simulink model "volo_radio_controller"  (Simulink 8.0)
settings: Solver=ode45  SolverMode=SingleTasking  StartTime=0.0  StopTime=1000  RelTol=1e-3
InitFcn:
  | volo_radio_controller_init
values from neighbouring files (symbols this model uses):
  cFI = fi(cMult, 1, 13, 11)    [volo_radio_controller_init.m]
  gFI = fi(gain, 1, 13, 11)    [volo_radio_controller_init.m]
  sFI = fi(sMult, 1, 13, 11)    [volo_radio_controller_init.m]
undefined symbols (not defined in the file or in its folder): gcbh, xlBlockLoadCallback, xlGetNormalizedPeriod, xlipgetpartsetting
libraries: xbsIndex_r4 x380, xbsEDKLib_r4 x1
(part 4 of 5)

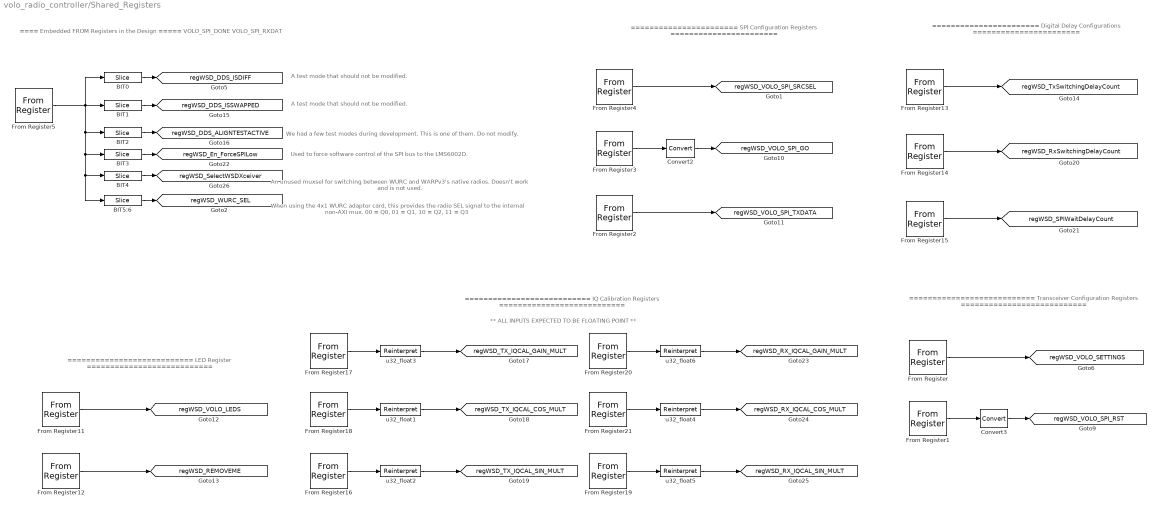
== system volo_radio_controller/Shared_Registers ==
  note: A test mode that should not be modified.
  note: We had a few test modes during development. This is one of them. Do not modify.
  note: Used to force software control of the SPI bus to the LMS6002D.
  note: When using the 4x1 WURC adaptor card, this provides the radio SEL signal
      | to the internal non-AXI mux.  00 = Q0, 01 = Q1, 10 = Q2, 11 = Q3
  note: An unused muxsel for switching between WURC and WARPv3's native radios.
      | Doesn't work and is not used.
  note: ==== Embedded FROM Registers in the Design =====
      | VOLO_SPI_DONE
      | VOLO_SPI_RXDAT
  note: ===========================
      | LED Register
      | ===========================
  note: =======================
      | Digital Delay Configurations
      | =======================
  note: =======================
      | SPI Configuration Registers
      | =======================
  note: ===========================
      | Transceiver Configuration Registers
      | ===========================
  note: ===========================
      | IQ Calibration Registers
      | ===========================
  note: ** ALL INPUTS EXPECTED TO BE FLOATING POINT **
  note: A test mode that should not be modified.
  BIT0 : xbsIndex_r4/Slice  nbits=1  boolean_output=on  mode=Lower Bit Location + Width  bit1=0  base1=LSB of Input  bit0=0  base0=LSB of Input  dbl_ovrd=off  block_type=slice
  BIT1 : xbsIndex_r4/Slice  nbits=1  boolean_output=on  mode=Lower Bit Location + Width  bit1=0  base1=LSB of Input  bit0=1  base0=LSB of Input  dbl_ovrd=off  block_type=slice
  BIT2 : xbsIndex_r4/Slice  nbits=1  boolean_output=on  mode=Lower Bit Location + Width  bit1=0  base1=LSB of Input  bit0=2  base0=LSB of Input  dbl_ovrd=off  block_type=slice
  BIT3 : xbsIndex_r4/Slice  nbits=1  boolean_output=on  mode=Lower Bit Location + Width  bit1=0  base1=LSB of Input  bit0=3  base0=LSB of Input  dbl_ovrd=off  block_type=slice
  BIT4 : xbsIndex_r4/Slice  nbits=1  boolean_output=on  mode=Lower Bit Location + Width  bit1=0  base1=LSB of Input  bit0=4  base0=LSB of Input  dbl_ovrd=off  block_type=slice
  BIT5:6 : xbsIndex_r4/Slice  nbits=2  boolean_output=off  mode=Lower Bit Location + Width  bit1=0  base1=LSB of Input  bit0=5  base0=LSB of Input  dbl_ovrd=off  block_type=slice
  Convert2 : xbsIndex_r4/Convert  gui_display_data_type=Boolean  arith_type=Boolean  n_bits=32  bin_pt=0  float_type=Single  exp_bits=8  fraction_bits=24  quantization=Truncate  overflow=Wrap  en=off  latency=0  dbl_ovrd=off  pipeline=off  block_type=convert
  Convert3 : xbsIndex_r4/Convert  gui_display_data_type=Boolean  arith_type=Boolean  n_bits=32  bin_pt=0  float_type=Single  exp_bits=8  fraction_bits=24  quantization=Truncate  overflow=Wrap  en=off  latency=0  dbl_ovrd=off  pipeline=off  block_type=convert
  From Register : xbsIndex_r4/From Register  shared_memory_name='VOLO_SETTINGS'  init=15  period=1  ownership=Locally owned and initialized  gui_display_data_type=Fixed-point  arith_type=Unsigned  n_bits=32  bin_pt=0  preci_type=Single  dbl_ovrd=off  block_type=fromreg
      settings: AttributesFormatString=<< %<shared_memory_name> >>  infoedit="Register block that reads data to a shared memory register.  Delay of one sample period."
  From Register1 : xbsIndex_r4/From Register  shared_memory_name='VOLO_SPI_RST'  init=0  period=1  ownership=Locally owned and initialized  gui_display_data_type=Fixed-point  arith_type=Unsigned  n_bits=1  bin_pt=0  preci_type=Single  dbl_ovrd=off  block_type=fromreg
      settings: AttributesFormatString=<< %<shared_memory_name> >>  infoedit="Register block that reads data to a shared memory register.  Delay of one sample period."
  From Register11 : xbsIndex_r4/From Register  shared_memory_name='VOLO_LED'  init=0  period=1  ownership=Owned and initialized elsewhere  gui_display_data_type=Fixed-point  arith_type=Unsigned  n_bits=32  bin_pt=0  preci_type=Single  dbl_ovrd=off  block_type=fromreg
      settings: AttributesFormatString=<< %<shared_memory_name> >>  infoedit="Register block that reads data to a shared memory register.  Delay of one sample period."
  From Register12 : xbsIndex_r4/From Register  shared_memory_name='VOLO_ADAPTER_GPIO'  init=0  period=1  ownership=Owned and initialized elsewhere  gui_display_data_type=Fixed-point  arith_type=Unsigned  n_bits=32  bin_pt=0  preci_type=Single  dbl_ovrd=off  block_type=fromreg
      settings: AttributesFormatString=<< %<shared_memory_name> >>  infoedit="Register block that reads data to a shared memory register.  Delay of one sample period."
  From Register13 : xbsIndex_r4/From Register  shared_memory_name='WSD_SWITCHINGDELAYCOUNT'  init=0  period=1  ownership=Locally owned and initialized  gui_display_data_type=Fixed-point  arith_type=Unsigned  n_bits=32  bin_pt=0  preci_type=Single  dbl_ovrd=off  block_type=fromreg
      settings: AttributesFormatString=<< %<shared_memory_name> >>  infoedit="Register block that reads data to a shared memory register.  Delay of one sample period."
  From Register14 : xbsIndex_r4/From Register  shared_memory_name='WSD_RXSWITCHINGDELAYCOUNT'  init=0  period=1  ownership=Locally owned and initialized  gui_display_data_type=Fixed-point  arith_type=Unsigned  n_bits=32  bin_pt=0  preci_type=Single  dbl_ovrd=off  block_type=fromreg
      settings: AttributesFormatString=<< %<shared_memory_name> >>  infoedit="Register block that reads data to a shared memory register.  Delay of one sample period."
  From Register15 : xbsIndex_r4/From Register  shared_memory_name='WSD_SPIWAITDELAYCOUNT'  init=0  period=1  ownership=Locally owned and initialized  gui_display_data_type=Fixed-point  arith_type=Unsigned  n_bits=32  bin_pt=0  preci_type=Single  dbl_ovrd=off  block_type=fromreg
      settings: AttributesFormatString=<< %<shared_memory_name> >>  infoedit="Register block that reads data to a shared memory register.  Delay of one sample period."
  From Register16 : xbsIndex_r4/From Register  shared_memory_name='VOLO_TX_SIN_MULT'  init=str2num(sFI.dec)  period=2  ownership=Locally owned and initialized  gui_display_data_type=Fixed-point  arith_type=Unsigned  n_bits=32  bin_pt=0  preci_type=Single  dbl_ovrd=off  block_type=fromreg
      settings: AttributesFormatString=<< %<shared_memory_name> >>  infoedit="Register block that reads data to a shared memory register.  Delay of one sample period."
  From Register17 : xbsIndex_r4/From Register  shared_memory_name='VOLO_TX_GAIN_MULT'  init=str2num(gFI.dec)  period=2  ownership=Locally owned and initialized  gui_display_data_type=Fixed-point  arith_type=Unsigned  n_bits=32  bin_pt=0  preci_type=Single  dbl_ovrd=off  block_type=fromreg
      settings: AttributesFormatString=<< %<shared_memory_name> >>  infoedit="Register block that reads data to a shared memory register.  Delay of one sample period."
  From Register18 : xbsIndex_r4/From Register  shared_memory_name='VOLO_TX_COS_MULT'  init=str2num(cFI.dec)  period=2  ownership=Locally owned and initialized  gui_display_data_type=Fixed-point  arith_type=Unsigned  n_bits=32  bin_pt=0  preci_type=Single  dbl_ovrd=off  block_type=fromreg
      settings: AttributesFormatString=<< %<shared_memory_name> >>  infoedit="Register block that reads data to a shared memory register.  Delay of one sample period."
  From Register19 : xbsIndex_r4/From Register  shared_memory_name='VOLO_RX_SIN_MULT'  init=str2num(sFI.dec)  period=2  ownership=Locally owned and initialized  gui_display_data_type=Fixed-point  arith_type=Unsigned  n_bits=32  bin_pt=0  preci_type=Single  dbl_ovrd=off  block_type=fromreg
      settings: AttributesFormatString=<< %<shared_memory_name> >>  infoedit="Register block that reads data to a shared memory register.  Delay of one sample period."
  From Register2 : xbsIndex_r4/From Register  shared_memory_name='VOLO_SPI_TXDAT'  init=hex2dec('ADAD')  period=1  ownership=Locally owned and initialized  gui_display_data_type=Fixed-point  arith_type=Unsigned  n_bits=32  bin_pt=0  preci_type=Single  dbl_ovrd=off  block_type=fromreg
      settings: AttributesFormatString=<< %<shared_memory_name> >>  infoedit="Register block that reads data to a shared memory register.  Delay of one sample period."
  From Register20 : xbsIndex_r4/From Register  shared_memory_name='VOLO_RX_GAIN_MULT'  init=str2num(gFI.dec)  period=2  ownership=Locally owned and initialized  gui_display_data_type=Fixed-point  arith_type=Unsigned  n_bits=32  bin_pt=0  preci_type=Single  dbl_ovrd=off  block_type=fromreg
      settings: AttributesFormatString=<< %<shared_memory_name> >>  infoedit="Register block that reads data to a shared memory register.  Delay of one sample period."
  From Register21 : xbsIndex_r4/From Register  shared_memory_name='VOLO_RX_COS_MULT'  init=str2num(cFI.dec)  period=2  ownership=Locally owned and initialized  gui_display_data_type=Fixed-point  arith_type=Unsigned  n_bits=32  bin_pt=0  preci_type=Single  dbl_ovrd=off  block_type=fromreg
      settings: AttributesFormatString=<< %<shared_memory_name> >>  infoedit="Register block that reads data to a shared memory register.  Delay of one sample period."
  From Register3 : xbsIndex_r4/From Register  shared_memory_name='VOLO_SPI_GO'  init=1  period=1  ownership=Locally owned and initialized  gui_display_data_type=Fixed-point  arith_type=Unsigned  n_bits=1  bin_pt=0  preci_type=Single  dbl_ovrd=off  block_type=fromreg
      settings: AttributesFormatString=<< %<shared_memory_name> >>  infoedit="Register block that reads data to a shared memory register.  Delay of one sample period."
  From Register4 : xbsIndex_r4/From Register  shared_memory_name='VOLO_SPI_SRCSEL'  init=1  period=1  ownership=Locally owned and initialized  gui_display_data_type=Fixed-point  arith_type=Unsigned  n_bits=1  bin_pt=0  preci_type=Single  dbl_ovrd=off  block_type=fromreg
      settings: AttributesFormatString=<< %<shared_memory_name> >>  infoedit="Register block that reads data to a shared memory register.  Delay of one sample period."
  From Register5 : xbsIndex_r4/From Register  shared_memory_name='VOLO_CONTROLLER_CONFIG_R'  init=19  period=1  ownership=Locally owned and initialized  gui_display_data_type=Fixed-point  arith_type=Unsigned  n_bits=32  bin_pt=0  preci_type=Single  dbl_ovrd=off  block_type=fromreg
      settings: AttributesFormatString=<< %<shared_memory_name> >>  infoedit="Register block that reads data to a shared memory register.  Delay of one sample period."
  u32_float{1..6} (6 alike) : xbsIndex_r4/Reinterpret  force_arith_type=on  arith_type=Floating-point  force_bin_pt=on  bin_pt=24  block_type=reinterpret
  tag scope: regWSD_DDS_ALIGNTESTACTIVE=global, regWSD_DDS_ISDIFF=global, regWSD_DDS_ISSWAPPED=global, regWSD_En_ForceSPILow=global, regWSD_REMOVEME=global, regWSD_RX_IQCAL_COS_MULT=global, regWSD_RX_IQCAL_GAIN_MULT=global, regWSD_RX_IQCAL_SIN_MULT=global, regWSD_RxSwitchingDelayCount=global, regWSD_SPIWaitDelayCount=global, regWSD_SelectWSDXceiver=global, regWSD_TX_IQCAL_COS_MULT=global, regWSD_TX_IQCAL_GAIN_MULT=global, regWSD_TX_IQCAL_SIN_MULT=global, regWSD_TxSwitchingDelayCount=global, regWSD_VOLO_LEDS=global, regWSD_VOLO_SETTINGS=global, regWSD_VOLO_SPI_GO=global, regWSD_VOLO_SPI_RST=global, regWSD_VOLO_SPI_SRCSEL=global, regWSD_VOLO_SPI_TXDATA=global, regWSD_WURC_SEL=global
  wires:
  From Register/1 -> [regWSD_VOLO_SETTINGS]
  From Register1/1 -> Convert3/1
  Convert3/1 -> [regWSD_VOLO_SPI_RST]
  From Register4/1 -> [regWSD_VOLO_SPI_SRCSEL]
  From Register3/1 -> Convert2/1
  Convert2/1 -> [regWSD_VOLO_SPI_GO]
  From Register2/1 -> [regWSD_VOLO_SPI_TXDATA]
  BIT0/1 -> [regWSD_DDS_ISDIFF]
  From Register11/1 -> [regWSD_VOLO_LEDS]
  From Register12/1 -> [regWSD_REMOVEME]
  From Register17/1 -> u32_float3/1
  From Register18/1 -> u32_float1/1
  From Register16/1 -> u32_float2/1
  u32_float3/1 -> [regWSD_TX_IQCAL_GAIN_MULT]
  u32_float1/1 -> [regWSD_TX_IQCAL_COS_MULT]
  u32_float2/1 -> [regWSD_TX_IQCAL_SIN_MULT]
  From Register13/1 -> [regWSD_TxSwitchingDelayCount]
  BIT1/1 -> [regWSD_DDS_ISSWAPPED]
  BIT2/1 -> [regWSD_DDS_ALIGNTESTACTIVE]
  From Register15/1 -> [regWSD_SPIWaitDelayCount]
  From Register14/1 -> [regWSD_RxSwitchingDelayCount]
  BIT3/1 -> [regWSD_En_ForceSPILow]
  From Register5/1 -> BIT0/1, BIT2/1, BIT5:6/1, BIT4/1, BIT3/1, BIT1/1
  From Register20/1 -> u32_float6/1
  From Register21/1 -> u32_float4/1
  From Register19/1 -> u32_float5/1
  u32_float6/1 -> [regWSD_RX_IQCAL_GAIN_MULT]
  u32_float4/1 -> [regWSD_RX_IQCAL_COS_MULT]
  u32_float5/1 -> [regWSD_RX_IQCAL_SIN_MULT]
  BIT4/1 -> [regWSD_SelectWSDXceiver]
  BIT5:6/1 -> [regWSD_WURC_SEL]

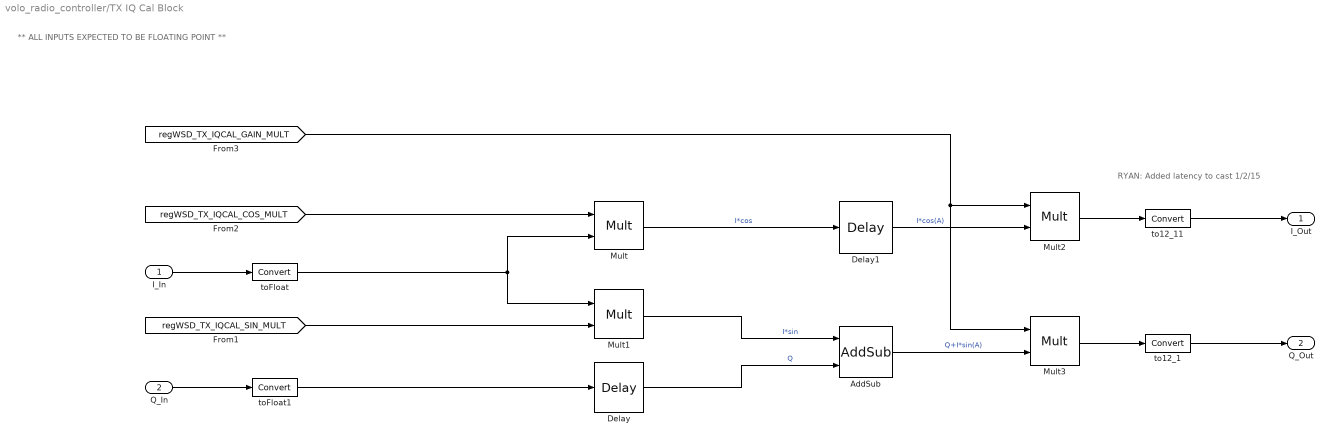
== system volo_radio_controller/TX IQ Cal Block ==
  note: RYAN: Added latency to cast 1/2/15
  note: ** ALL INPUTS EXPECTED TO BE FLOATING POINT **
  I_In : Inport
  Q_In : Inport  Port=2
  AddSub : xbsIndex_r4/AddSub  mode=Addition  use_carryin=off  use_carryout=off  en=off  latency=1  precision=Full  arith_type="Signed  (2's comp)"  n_bits=13  bin_pt=11  quantization="Round  (unbiased: +/- Inf)"  overflow=Flag as error  dbl_ovrd=off  use_behavioral_HDL=off  hw_selection=Fabric  pipelined=off  block_type=addsub
  Delay : xbsIndex_r4/Delay  rst=off  infoeditControl=Selection of Reset will increase slice count due to use of real FFs and instead of SRLs  en=off  latency=3  dbl_ovrd=off  reg_retiming=off  block_type=delay
  Delay1 : xbsIndex_r4/Delay  rst=off  infoeditControl=Selection of Reset will increase slice count due to use of real FFs and instead of SRLs  en=off  latency=1  dbl_ovrd=off  reg_retiming=off  block_type=delay
  Mult : xbsIndex_r4/Mult  precision=Full  arith_type="Signed  (2's comp)"  n_bits=13  bin_pt=11  quantization="Round  (unbiased: +/- Inf)"  overflow=Saturate  en=off  latency=3  dbl_ovrd=off  use_behavioral_HDL=off  opt=Speed  use_embedded=on  optimum_pipeline=off  pipeline=on  use_rpm=on  placement_style=Triangular  block_type=mult
  Mult1 : xbsIndex_r4/Mult  precision=Full  arith_type="Signed  (2's comp)"  n_bits=13  bin_pt=11  quantization="Round  (unbiased: +/- Inf)"  overflow=Saturate  en=off  latency=3  dbl_ovrd=off  use_behavioral_HDL=off  opt=Speed  use_embedded=on  optimum_pipeline=off  pipeline=on  use_rpm=on  placement_style=Triangular  block_type=mult
  Mult2 : xbsIndex_r4/Mult  precision=Full  arith_type="Signed  (2's comp)"  n_bits=12  bin_pt=11  quantization="Round  (unbiased: +/- Inf)"  overflow=Flag as error  en=off  latency=3  dbl_ovrd=off  use_behavioral_HDL=off  opt=Speed  use_embedded=on  optimum_pipeline=off  pipeline=on  use_rpm=on  placement_style=Triangular  block_type=mult
  Mult3 : xbsIndex_r4/Mult  precision=Full  arith_type="Signed  (2's comp)"  n_bits=12  bin_pt=11  quantization="Round  (unbiased: +/- Inf)"  overflow=Saturate  en=off  latency=3  dbl_ovrd=off  use_behavioral_HDL=off  opt=Speed  use_embedded=on  optimum_pipeline=off  pipeline=on  use_rpm=on  placement_style=Triangular  block_type=mult
  to12_1 : xbsIndex_r4/Convert  gui_display_data_type=Fixed-point  arith_type="Signed  (2's comp)"  n_bits=12  bin_pt=11  float_type=Single  exp_bits=8  fraction_bits=24  quantization="Round  (unbiased: +/- Inf)"  overflow=Saturate  en=off  latency=1  dbl_ovrd=off  pipeline=off  block_type=convert
  to12_11 : xbsIndex_r4/Convert  gui_display_data_type=Fixed-point  arith_type="Signed  (2's comp)"  n_bits=12  bin_pt=11  float_type=Single  exp_bits=8  fraction_bits=24  quantization="Round  (unbiased: +/- Inf)"  overflow=Saturate  en=off  latency=1  dbl_ovrd=off  pipeline=off  block_type=convert
  toFloat : xbsIndex_r4/Convert  gui_display_data_type=Floating-point  arith_type=Floating-point  n_bits=13  bin_pt=11  float_type=Single  exp_bits=8  fraction_bits=24  quantization="Round  (unbiased: +/- Inf)"  overflow=Flag as error  en=off  latency=0  dbl_ovrd=off  pipeline=off  block_type=convert
  toFloat1 : xbsIndex_r4/Convert  gui_display_data_type=Floating-point  arith_type=Floating-point  n_bits=13  bin_pt=11  float_type=Single  exp_bits=8  fraction_bits=24  quantization="Round  (unbiased: +/- Inf)"  overflow=Flag as error  en=off  latency=0  dbl_ovrd=off  pipeline=off  block_type=convert
  I_Out : Outport
  Q_Out : Outport  Port=2
  wires:
  I_In/1 -> toFloat/1
  [regWSD_TX_IQCAL_COS_MULT] -> Mult/1
  Q_In/1 -> toFloat1/1
  Mult/1 -> Delay1/1  "I*cos"
  Mult1/1 -> AddSub/1  "I*sin"
  [regWSD_TX_IQCAL_GAIN_MULT] -> Mult3/1, Mult2/1
  Mult2/1 -> to12_11/1
  Mult3/1 -> to12_1/1
  Delay1/1 -> Mult2/2  "I*cos(A)"
  AddSub/1 -> Mult3/2  "Q+I*sin(A)"
  Delay/1 -> AddSub/2  "Q"
  [regWSD_TX_IQCAL_SIN_MULT] -> Mult1/2
  toFloat/1 -> Mult/2, Mult1/1
  toFloat1/1 -> Delay/1
  to12_11/1 -> I_Out/1
  to12_1/1 -> Q_Out/1

== system volo_radio_controller/TX_MUXes ==
  note: 00 - MyDDS
      | 01 - External
      | 10 - RX LoopBack
      | 11 - RX_Proccessed_Loopback
  MUXSEL : Inport
  DDS_I : Inport  Port=2
  BB_I : Inport  Port=3
  RX_I : Inport  Port=4
  ZERO_I : Inport  Port=5
  DDS_Q : Inport  Port=6
  BB_Q : Inport  Port=7
  RX_Q : Inport  Port=8
  ZERO_Q : Inport  Port=9
  Mux : xbsIndex_r4/Mux  inputs=4  en=off  latency=0  precision=Full  arith_type=Unsigned  n_bits=16  bin_pt=14  quantization=Truncate  overflow=Wrap  dbl_ovrd=off  block_type=mux
      settings: xl_area=[6 0 0 12 0 0 0]
  Mux1 : xbsIndex_r4/Mux  inputs=4  en=off  latency=0  precision=Full  arith_type=Unsigned  n_bits=16  bin_pt=14  quantization=Truncate  overflow=Wrap  dbl_ovrd=off  block_type=mux
      settings: xl_area=[6 0 0 12 0 0 0]
  TXI : Outport
  TXQ : Outport  Port=2
  wires:
  Mux/1 -> TXI/1
  Mux1/1 -> TXQ/1
  DDS_I/1 -> Mux/2
  DDS_Q/1 -> Mux1/2
  MUXSEL/1 -> Mux/1, Mux1/1
  BB_I/1 -> Mux/3
  BB_Q/1 -> Mux1/3
  RX_Q/1 -> Mux1/4
  ZERO_Q/1 -> Mux1/5
  RX_I/1 -> Mux/4
  ZERO_I/1 -> Mux/5

== system volo_radio_controller/UART Controller ==
  note: This signal passthrough is performed so that every I/O from the WSD comes through the radio controller.
      | This makes a bit more sense in my head, I hope it does yours.
  Terminator1 : Terminator
  Terminator7 : Terminator
  UART_RX : xbsIndex_r4/Gateway Out  inherit_from_input=off  hdl_port=on  timing_constraint=None  locs_specified=off  LOCs={}  UseAsDAC=off  DACChannel='1'  block_type=gatewayout
      settings: infoedit="Gateway out block.  Converts Xilinx fixed-point or floating-point type inputs into ouputs of type Simulink integer, single, double, or fixed point.<br><br>Hardware notes:  In hardware these blocks become top level output ports or are discarded, depending on how they are configured."  xl_area=[0 0 0 0 1 0 0]
  UART_RX_UBLAZE : xbsIndex_r4/Gateway Out  inherit_from_input=off  hdl_port=on  timing_constraint=None  locs_specified=off  LOCs={}  UseAsDAC=off  DACChannel='1'  block_type=gatewayout
      settings: infoedit="Gateway out block.  Converts Xilinx fixed-point or floating-point type inputs into ouputs of type Simulink integer, single, double, or fixed point.<br><br>Hardware notes:  In hardware these blocks become top level output ports or are discarded, depending on how they are configured."  xl_area=[0 0 0 0 1 0 0]
  UART_TX : xbsIndex_r4/Gateway In  gui_display_data_type=Boolean  arith_type=Boolean  n_bits=1  bin_pt=0  preci_type=Single  exp_width=8  frac_width=24  quantization=Truncate  overflow=Saturate  period=1  dbl_ovrd=off  timing_constraint=None  locs_specified=off  LOCs={}  UseAsADC=off  ADCChannel='1'  inherit_from_input=off  hdl_port=on  block_type=gatewayin
      settings: xl_area=[0 0 0 0 1 0 0]
  UART_TX_UBLAZE : xbsIndex_r4/Gateway In  gui_display_data_type=Boolean  arith_type=Boolean  n_bits=16  bin_pt=14  preci_type=Single  exp_width=8  frac_width=24  quantization="Round  (unbiased: +/- Inf)"  overflow=Saturate  period=1  dbl_ovrd=off  timing_constraint=None  locs_specified=off  LOCs={}  UseAsADC=off  ADCChannel='1'  inherit_from_input=off  hdl_port=on  block_type=gatewayin
      settings: xl_area=[0 0 0 0 1 0 0]
  wires:
  UART_RX/1 -> Terminator7/1
  UART_TX_UBLAZE/1 -> UART_RX/1
  UART_TX/1 -> UART_RX_UBLAZE/1
  UART_RX_UBLAZE/1 -> Terminator1/1

== system volo_radio_controller/UNUSED Radio IO Ports ==
  note: Output to Stellaris
  TieLow : xbsIndex_r4/Constant  const=0  gui_display_data_type=Fixed-point  arith_type=Unsigned  n_bits=1  bin_pt=0  preci_type=Single  exp_width=8  frac_width=24  explicit_period=off  period=1  equ=P=C  opselect=C  inp2=PCIN>>17  opr=+  inp1=P  carry=CIN  dbl_ovrd=off  block_type=constant
  uC_NMI : xbsIndex_r4/Gateway Out  inherit_from_input=off  hdl_port=on  timing_constraint=None  locs_specified=off  LOCs={}  UseAsDAC=off  DACChannel='1'  block_type=gatewayout
      settings: infoedit="Gateway out block.  Converts Xilinx fixed-point or floating-point type inputs into ouputs of type Simulink integer, single, double, or fixed point.<br><br>Hardware notes:  In hardware these blocks become top level output ports or are discarded, depending on how they are configured."  xl_area=[0 0 0 0 1 0 0]
  wires:
  TieLow/1 -> uC_NMI/1

== system volo_radio_controller/Digital Synthesizer/Square Wave Generator ==
  Constant : xbsIndex_r4/Constant  const=0.8  gui_display_data_type=Fixed-point  arith_type=Signed (2's comp)  n_bits=12  bin_pt=11  preci_type=Single  exp_width=8  frac_width=24  explicit_period=off  period=1  equ=P=C  opselect=C  inp2=PCIN>>17  opr=+  inp1=P  carry=CIN  dbl_ovrd=off  block_type=constant
  Constant1 : xbsIndex_r4/Constant  const=-0.8  gui_display_data_type=Fixed-point  arith_type=Signed (2's comp)  n_bits=12  bin_pt=11  preci_type=Single  exp_width=8  frac_width=24  explicit_period=off  period=1  equ=P=C  opselect=C  inp2=PCIN>>17  opr=+  inp1=P  carry=CIN  dbl_ovrd=off  block_type=constant
  Counter : xbsIndex_r4/Counter  cnt_type=Free Running  cnt_to=Inf  operation=Up  start_count=0  cnt_by_val=1  arith_type=Unsigned  n_bits=1  bin_pt=0  load_pin=off  rst=off  en=off  explicit_period=on  period=1  dbl_ovrd=off  use_behavioral_HDL=off  implementation=Fabric  block_type=counter
      settings: xl_area=[2 1 0 1 0 0 0]
  Mux5 : xbsIndex_r4/Mux  inputs=2  en=off  latency=1  precision=Full  arith_type=Unsigned  n_bits=16  bin_pt=14  quantization=Truncate  overflow=Wrap  dbl_ovrd=off  block_type=mux
      settings: xl_area=[6 12 0 12 0 0 0]
  Out : Outport
  wires:
  Constant/1 -> Mux5/2
  Counter/1 -> Mux5/1
  Mux5/1 -> Out/1
  Constant1/1 -> Mux5/3

== system volo_radio_controller/Digital Synthesizer/Square Wave Generator1 ==
  Constant : xbsIndex_r4/Constant  const=0.8  gui_display_data_type=Fixed-point  arith_type=Signed (2's comp)  n_bits=12  bin_pt=11  preci_type=Single  exp_width=8  frac_width=24  explicit_period=off  period=1  equ=P=C  opselect=C  inp2=PCIN>>17  opr=+  inp1=P  carry=CIN  dbl_ovrd=off  block_type=constant
  Constant1 : xbsIndex_r4/Constant  const=-0.8  gui_display_data_type=Fixed-point  arith_type=Signed (2's comp)  n_bits=12  bin_pt=11  preci_type=Single  exp_width=8  frac_width=24  explicit_period=off  period=1  equ=P=C  opselect=C  inp2=PCIN>>17  opr=+  inp1=P  carry=CIN  dbl_ovrd=off  block_type=constant
  Counter : xbsIndex_r4/Counter  cnt_type=Free Running  cnt_to=Inf  operation=Up  start_count=0  cnt_by_val=1  arith_type=Unsigned  n_bits=1  bin_pt=0  load_pin=off  rst=off  en=off  explicit_period=on  period=1  dbl_ovrd=off  use_behavioral_HDL=off  implementation=Fabric  block_type=counter
      settings: xl_area=[2 1 0 1 0 0 0]
  Mux5 : xbsIndex_r4/Mux  inputs=2  en=off  latency=1  precision=Full  arith_type=Unsigned  n_bits=16  bin_pt=14  quantization=Truncate  overflow=Wrap  dbl_ovrd=off  block_type=mux
      settings: xl_area=[6 12 0 12 0 0 0]
  Out : Outport
  wires:
  Constant/1 -> Mux5/3
  Counter/1 -> Mux5/1
  Mux5/1 -> Out/1
  Constant1/1 -> Mux5/2

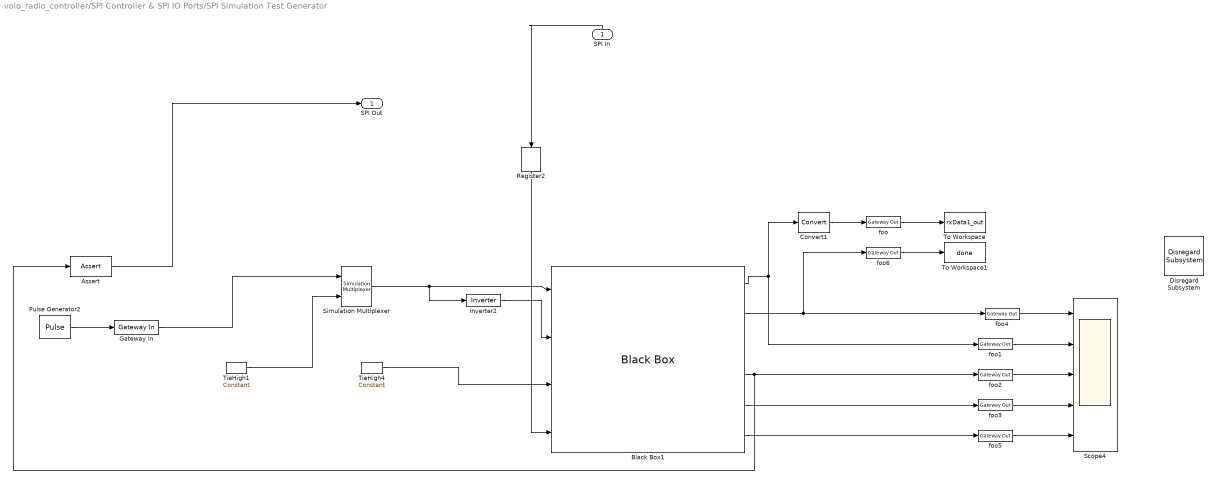
== system volo_radio_controller/SPI Controller & SPI IO Ports/SPI Simulation Test Generator ==
  SPI In : Inport
  Assert : xbsIndex_r4/Assert  assert_type=off  type_source=Explicitly  gui_display_data_type=Fixed-point  arith_type="Signed  (2's comp)"  n_bits=16  bin_pt=14  preci_type=Single  exp_width=8  frac_width=24  assert_rate=on  rate_source=Explicitly  period=1  output_port=on  block_type=assert
  Black Box1 : xbsIndex_r4/Black Box  init_code=volo_spi_io_config  sim_method=ISE Simulator  verbose=off  block_type=blackbox2
  Convert1 : xbsIndex_r4/Convert  gui_display_data_type=Fixed-point  arith_type=Unsigned  n_bits=32  bin_pt=0  float_type=Single  exp_bits=8  fraction_bits=24  quantization=Truncate  overflow=Wrap  en=off  latency=0  dbl_ovrd=off  pipeline=off  block_type=convert
  Disregard Subsystem : xbsIndex_r4/Disregard Subsystem  Tag=discardX  block_type=disregard
  Gateway In : xbsIndex_r4/Gateway In  gui_display_data_type=Boolean  arith_type=Boolean  n_bits=16  bin_pt=14  preci_type=Single  exp_width=8  frac_width=24  quantization="Round  (unbiased: +/- Inf)"  overflow=Saturate  period=1  dbl_ovrd=off  timing_constraint=None  locs_specified=off  LOCs={}  UseAsADC=off  ADCChannel='1'  inherit_from_input=off  hdl_port=on  block_type=gatewayin
  Inverter2 : xbsIndex_r4/Inverter  en=off  latency=0  dbl_ovrd=off  block_type=inv
  Pulse Generator2 : DiscretePulseGenerator  Period=5000  PhaseDelay=5
  Register2 : xbsIndex_r4/Register  init=0  rst=off  en=off  dbl_ovrd=off  block_type=register
      settings: xl_area=[6 12 0 0 0 0 0]  block_version=8.2
  Scope4 : Scope  NumInputPorts=5
      settings: YMin=-5~-5~-5~-5~-5  YMax=5~5~5~5~5  SaveName=ScopeData3
  Simulation Multiplexer : xbsIndex_r4/Simulation Multiplexer  sim_sel=1  hw_sel=2  block_type=simmux
      settings: infoedit="Distinguish input subsystems as \"simulation only\" and \"generation only\".  The input specified For Simulation will be used during Simulink simulation.  The input specified For Generation will be used during code generation.  This block will typically be used on the output of a HW Co-Simulation, Black Box, or ModelSim subsystem.<br><br>Hardware Notes: This block costs nothing."
  TieHigh1 : xbsIndex_r4/Constant  const=0  gui_display_data_type=Boolean  arith_type=Boolean  n_bits=3  bin_pt=0  preci_type=Single  exp_width=8  frac_width=24  explicit_period=on  period=1  equ=P=C  opselect=C  inp2=PCIN>>17  opr=+  inp1=P  carry=CIN  dbl_ovrd=off  block_type=constant
  TieHigh4 : xbsIndex_r4/Constant  const=hex2dec('CD')  gui_display_data_type=Fixed-point  arith_type=Unsigned  n_bits=32  bin_pt=0  preci_type=Single  exp_width=8  frac_width=24  explicit_period=on  period=1  equ=P=C  opselect=C  inp2=PCIN>>17  opr=+  inp1=P  carry=CIN  dbl_ovrd=off  block_type=constant
  To Workspace : ToWorkspace  VariableName=rxData1_out  SampleTime=-1
  To Workspace1 : ToWorkspace  VariableName=done  SampleTime=-1
  foo{,1..6} (7 alike) : xbsIndex_r4/Gateway Out  inherit_from_input=off  hdl_port=off  timing_constraint=None  locs_specified=off  LOCs={}  UseAsDAC=off  DACChannel='1'  block_type=gatewayout
      settings: xl_area=[0 0 0 0 1 0 0]
  SPI Out : Outport
  wires:
  Assert/1 -> SPI Out/1
  Black Box1/4 -> Assert/1, foo2/1
  Black Box1/6 -> foo5/1
  Black Box1/2 -> foo6/1, foo4/1
  SPI In/1 -> Register2/1
  Pulse Generator2/1 -> Gateway In/1
  Inverter2/1 -> Black Box1/2
  Black Box1/1 -> foo1/1, Convert1/1
  Black Box1/5 -> foo3/1
  Convert1/1 -> foo/1
  foo4/1 -> Scope4/1
  foo1/1 -> Scope4/2
  foo2/1 -> Scope4/3
  foo3/1 -> Scope4/4
  foo5/1 -> Scope4/5
  foo/1 -> To Workspace/1
  foo6/1 -> To Workspace1/1
  Simulation Multiplexer/1 -> Inverter2/1, Black Box1/1
  TieHigh1/1 -> Simulation Multiplexer/2
  Gateway In/1 -> Simulation Multiplexer/1
  TieHigh4/1 -> Black Box1/3
  Register2/1 -> Black Box1/4

== system volo_radio_controller/SPI Controller & SPI IO Ports/Simulation Input Generator ==
  Delay : xbsIndex_r4/Delay  rst=off  infoeditControl=Selection of Reset will increase slice count due to use of real FFs and instead of SRLs  en=off  latency=0  dbl_ovrd=off  reg_retiming=off  block_type=delay
  Disregard Subsystem : xbsIndex_r4/Disregard Subsystem  Tag=discardX  block_type=disregard
  Gateway In : xbsIndex_r4/Gateway In  gui_display_data_type=Boolean  arith_type=Boolean  n_bits=16  bin_pt=14  preci_type=Single  exp_width=8  frac_width=24  quantization="Round  (unbiased: +/- Inf)"  overflow=Saturate  period=1  dbl_ovrd=off  timing_constraint=None  locs_specified=off  LOCs={}  UseAsADC=off  ADCChannel='1'  inherit_from_input=off  hdl_port=on  block_type=gatewayin
  Pulse Generator1 : DiscretePulseGenerator  Period=5000  PhaseDelay=5
  Register2 : xbsIndex_r4/Register  init=1  rst=off  en=on  dbl_ovrd=off  block_type=register
      settings: xl_area=[6 12 0 0 0 0 0]  block_version=8.2
  Scope3 : Scope  NumInputPorts=2
      settings: YMin=-5~-5  YMax=5~5
  TieHigh1 : xbsIndex_r4/Constant  const=0  gui_display_data_type=Boolean  arith_type=Boolean  n_bits=1  bin_pt=0  preci_type=Single  exp_width=8  frac_width=24  explicit_period=on  period=1  equ=P=C  opselect=C  inp2=PCIN>>17  opr=+  inp1=P  carry=CIN  dbl_ovrd=off  block_type=constant
  foo1 : xbsIndex_r4/Gateway Out  inherit_from_input=off  hdl_port=off  timing_constraint=None  locs_specified=off  LOCs={}  UseAsDAC=off  DACChannel='1'  block_type=gatewayout
      settings: xl_area=[0 0 0 0 1 0 0]
  foo4 : xbsIndex_r4/Gateway Out  inherit_from_input=off  hdl_port=off  timing_constraint=None  locs_specified=off  LOCs={}  UseAsDAC=off  DACChannel='1'  block_type=gatewayout
      settings: xl_area=[0 0 0 0 1 0 0]
  Rst : Outport
  Go : Outport  Port=2
  wires:
  Pulse Generator1/1 -> Gateway In/1
  Gateway In/1 -> foo4/1, Rst/1
  foo4/1 -> Scope3/1
  foo1/1 -> Scope3/2
  Register2/1 -> Delay/1
  TieHigh1/1 -> Register2/1
  [SPI_DONE] -> Register2/2
  Delay/1 -> foo1/1, Go/1

== system volo_radio_controller/SPI Controller & SPI IO Ports/posedge1 ==
  D : Inport
  Delay : xbsIndex_r4/Delay  rst=off  infoeditControl=Selection of Reset will increase slice count due to use of real FFs and instead of SRLs  en=off  latency=1  dbl_ovrd=off  reg_retiming=off  block_type=delay
      settings: infoedit=Hardware notes: A delay line is a chain, each link of which is an SRL16 followed by a flip-flop. If register retiming is enabled, the delay line is a chain of flip-flops.  xl_area=[1 1 0 0 0 0 0]  block_version=VER_STRING_GOES_HERE
  Inverter : xbsIndex_r4/Inverter  en=off  latency=0  dbl_ovrd=off  block_type=inv
      settings: xl_area=[0 0 0 0 0 0 0]  block_version=VER_STRING_GOES_HERE
  Logical1 : xbsIndex_r4/Logical  logical_function=AND  inputs=2  en=off  latency=0  precision=Full  arith_type=Unsigned  n_bits=8  bin_pt=2  align_bp=on  dbl_ovrd=off  block_type=logical
      settings: xl_area=[1 0 0 1 0 0 0]  block_version=VER_STRING_GOES_HERE
  Q : Outport
  wires:
  Inverter/1 -> Logical1/1
  D/1 -> Logical1/2, Delay/1
  Delay/1 -> Inverter/1
  Logical1/1 -> Q/1

== system volo_radio_controller/Shared Registers and IO Ports/RX Switching Delay ==
  note: Note: If the input value changes at any time while the oneshot is
      | counting, it will be reset and Out will never change state
  note: Note: 32-bit count value gives you up to 53-second delay with a 80 MHz clock.
      | (2^32-1)/80e6 = 53.7 sec
  In : Inport
  32Bit_OneShot : Subsystem
  Inverter : xbsIndex_r4/Inverter  en=off  latency=0  dbl_ovrd=off  block_type=inv
  Logical : xbsIndex_r4/Logical  logical_function=XOR  inputs=2  en=off  latency=0  precision=Full  arith_type=Unsigned  n_bits=16  bin_pt=0  align_bp=on  dbl_ovrd=off  block_type=logical
  Old Configurable Delay Block : Subsystem  Commented=on
  Register : xbsIndex_r4/Register  init=0  rst=off  en=on  dbl_ovrd=off  block_type=register
  rising edge : Subsystem
  Out : Outport
  wires:
  In/1 -> Register/1, Logical/2  "input"
  Logical/1 -> 32Bit_OneShot/1(Start), Inverter/1  "output unsynched"
  [regWSD_RxSwitchingDelayCount] -> 32Bit_OneShot/2(CountTo)
  32Bit_OneShot/1(Done) -> rising edge/1(A)
  Inverter/1 -> 32Bit_OneShot/3(RST)  "output synched"
  rising edge/1(Q) -> Register/2
  Register/1 -> Logical/1, Out/1  "output"

== system volo_radio_controller/Shared Registers and IO Ports/S-R Latch1 ==
  S : Inport
  R : Inport  Port=2
  Constant1 : xbsIndex_r4/Constant  const=1  gui_display_data_type=Fixed-point  arith_type=Boolean  n_bits=1  bin_pt=0  preci_type=Single  exp_width=8  frac_width=24  explicit_period=off  period=1  equ=P=C  opselect=C  inp2=PCIN>>17  opr=+  inp1=P  carry=CIN  dbl_ovrd=off  block_type=constant
      settings: block_version=VER_STRING_GOES_HERE
  Convert : xbsIndex_r4/Convert  gui_display_data_type=Fixed-point  arith_type=Boolean  n_bits=16  bin_pt=14  float_type=Single  exp_bits=8  fraction_bits=24  quantization=Truncate  overflow=Wrap  en=off  latency=0  dbl_ovrd=off  pipeline=off  block_type=convert
      settings: block_version=10.1.3
  Convert1 : xbsIndex_r4/Convert  gui_display_data_type=Fixed-point  arith_type=Boolean  n_bits=16  bin_pt=14  float_type=Single  exp_bits=8  fraction_bits=24  quantization=Truncate  overflow=Wrap  en=off  latency=0  dbl_ovrd=off  pipeline=off  block_type=convert
      settings: block_version=10.1.3
  Register2 : xbsIndex_r4/Register  init=0  rst=on  en=on  dbl_ovrd=off  block_type=register
      settings: xl_area=[1 1 0 0 0 0 0]  block_version=VER_STRING_GOES_HERE
  Q : Outport
  wires:
  Convert1/1 -> Register2/3
  Convert/1 -> Register2/2
  S/1 -> Convert1/1
  Register2/1 -> Q/1
  R/1 -> Convert/1
  Constant1/1 -> Register2/1

== system volo_radio_controller/Shared Registers and IO Ports/S-R Latch2 ==
  S : Inport
  R : Inport  Port=2
  Constant1 : xbsIndex_r4/Constant  const=1  gui_display_data_type=Fixed-point  arith_type=Boolean  n_bits=1  bin_pt=0  preci_type=Single  exp_width=8  frac_width=24  explicit_period=off  period=1  equ=P=C  opselect=C  inp2=PCIN>>17  opr=+  inp1=P  carry=CIN  dbl_ovrd=off  block_type=constant
      settings: block_version=VER_STRING_GOES_HERE
  Convert : xbsIndex_r4/Convert  gui_display_data_type=Fixed-point  arith_type=Boolean  n_bits=16  bin_pt=14  float_type=Single  exp_bits=8  fraction_bits=24  quantization=Truncate  overflow=Wrap  en=off  latency=0  dbl_ovrd=off  pipeline=off  block_type=convert
      settings: block_version=10.1.3
  Convert1 : xbsIndex_r4/Convert  gui_display_data_type=Fixed-point  arith_type=Boolean  n_bits=16  bin_pt=14  float_type=Single  exp_bits=8  fraction_bits=24  quantization=Truncate  overflow=Wrap  en=off  latency=0  dbl_ovrd=off  pipeline=off  block_type=convert
      settings: block_version=10.1.3
  Register2 : xbsIndex_r4/Register  init=0  rst=on  en=on  dbl_ovrd=off  block_type=register
      settings: xl_area=[1 1 0 0 0 0 0]  block_version=VER_STRING_GOES_HERE
  Q : Outport
  wires:
  Convert1/1 -> Register2/3
  Convert/1 -> Register2/2
  S/1 -> Convert1/1
  Register2/1 -> Q/1
  R/1 -> Convert/1
  Constant1/1 -> Register2/1

== system volo_radio_controller/Shared Registers and IO Ports/S-R Latch3 ==
  S : Inport
  R : Inport  Port=2
  Constant1 : xbsIndex_r4/Constant  const=1  gui_display_data_type=Fixed-point  arith_type=Boolean  n_bits=1  bin_pt=0  preci_type=Single  exp_width=8  frac_width=24  explicit_period=off  period=1  equ=P=C  opselect=C  inp2=PCIN>>17  opr=+  inp1=P  carry=CIN  dbl_ovrd=off  block_type=constant
      settings: block_version=VER_STRING_GOES_HERE
  Convert : xbsIndex_r4/Convert  gui_display_data_type=Fixed-point  arith_type=Boolean  n_bits=16  bin_pt=14  float_type=Single  exp_bits=8  fraction_bits=24  quantization=Truncate  overflow=Wrap  en=off  latency=0  dbl_ovrd=off  pipeline=off  block_type=convert
      settings: block_version=10.1.3
  Convert1 : xbsIndex_r4/Convert  gui_display_data_type=Fixed-point  arith_type=Boolean  n_bits=16  bin_pt=14  float_type=Single  exp_bits=8  fraction_bits=24  quantization=Truncate  overflow=Wrap  en=off  latency=0  dbl_ovrd=off  pipeline=off  block_type=convert
      settings: block_version=10.1.3
  Register2 : xbsIndex_r4/Register  init=0  rst=on  en=on  dbl_ovrd=off  block_type=register
      settings: xl_area=[1 1 0 0 0 0 0]  block_version=VER_STRING_GOES_HERE
  Q : Outport
  wires:
  Convert1/1 -> Register2/3
  Convert/1 -> Register2/2
  S/1 -> Convert1/1
  Register2/1 -> Q/1
  R/1 -> Convert/1
  Constant1/1 -> Register2/1

== system volo_radio_controller/Shared Registers and IO Ports/S-R Latch4 ==
  S : Inport
  R : Inport  Port=2
  Constant1 : xbsIndex_r4/Constant  const=1  gui_display_data_type=Fixed-point  arith_type=Boolean  n_bits=1  bin_pt=0  preci_type=Single  exp_width=8  frac_width=24  explicit_period=off  period=1  equ=P=C  opselect=C  inp2=PCIN>>17  opr=+  inp1=P  carry=CIN  dbl_ovrd=off  block_type=constant
      settings: block_version=VER_STRING_GOES_HERE
  Convert : xbsIndex_r4/Convert  gui_display_data_type=Fixed-point  arith_type=Boolean  n_bits=16  bin_pt=14  float_type=Single  exp_bits=8  fraction_bits=24  quantization=Truncate  overflow=Wrap  en=off  latency=0  dbl_ovrd=off  pipeline=off  block_type=convert
      settings: block_version=10.1.3
  Convert1 : xbsIndex_r4/Convert  gui_display_data_type=Fixed-point  arith_type=Boolean  n_bits=16  bin_pt=14  float_type=Single  exp_bits=8  fraction_bits=24  quantization=Truncate  overflow=Wrap  en=off  latency=0  dbl_ovrd=off  pipeline=off  block_type=convert
      settings: block_version=10.1.3
  Register2 : xbsIndex_r4/Register  init=0  rst=on  en=on  dbl_ovrd=off  block_type=register
      settings: xl_area=[1 1 0 0 0 0 0]  block_version=VER_STRING_GOES_HERE
  Q : Outport
  wires:
  Constant1/1 -> Register2/1
  R/1 -> Convert/1
  Register2/1 -> Q/1
  S/1 -> Convert1/1
  Convert/1 -> Register2/2
  Convert1/1 -> Register2/3

== system volo_radio_controller/Shared Registers and IO Ports/SPI Flush Delay  ==
  note: Note: If the input value changes at any time while the oneshot is
      | counting, it will be reset and Out will never change state
  In : Inport
  32Bit_OneShot : Subsystem
  Inverter : xbsIndex_r4/Inverter  en=off  latency=0  dbl_ovrd=off  block_type=inv
  Logical : xbsIndex_r4/Logical  logical_function=XOR  inputs=2  en=off  latency=0  precision=Full  arith_type=Unsigned  n_bits=16  bin_pt=0  align_bp=on  dbl_ovrd=off  block_type=logical
  Old Configurable Delay Block : Subsystem  Commented=on
  Register : xbsIndex_r4/Register  init=0  rst=off  en=on  dbl_ovrd=off  block_type=register
  rising edge : Subsystem
  Out : Outport
  wires:
  In/1 -> Register/1, Logical/2  "input"
  Logical/1 -> 32Bit_OneShot/1(Start), Inverter/1  "output unsynched"
  [regWSD_SPIWaitDelayCount] -> 32Bit_OneShot/2(CountTo)
  32Bit_OneShot/1(Done) -> rising edge/1(A)
  Inverter/1 -> 32Bit_OneShot/3(RST)  "output synched"
  rising edge/1(Q) -> Register/2
  Register/1 -> Logical/1, Out/1  "output"

== system volo_radio_controller/Shared Registers and IO Ports/TX Switching Delay ==
  note: Note: If the input value changes at any time while the oneshot is
      | counting, it will be reset and Out will never change state
  note: Note: 32-bit count value gives you up to 53-second delay with a 80 MHz clock.
      | (2^32-1)/80e6 = 53.7 sec
  In : Inport
  32Bit_OneShot : Subsystem
  Inverter : xbsIndex_r4/Inverter  en=off  latency=0  dbl_ovrd=off  block_type=inv
  Logical : xbsIndex_r4/Logical  logical_function=XOR  inputs=2  en=off  latency=0  precision=Full  arith_type=Unsigned  n_bits=16  bin_pt=0  align_bp=on  dbl_ovrd=off  block_type=logical
  Old Configurable Delay Block : Subsystem  Commented=on
  Register : xbsIndex_r4/Register  init=0  rst=off  en=on  dbl_ovrd=off  block_type=register
  rising edge : Subsystem
  Out : Outport
  wires:
  In/1 -> Register/1, Logical/2  "input"
  Logical/1 -> 32Bit_OneShot/1(Start), Inverter/1  "output unsynched"
  [regWSD_TxSwitchingDelayCount] -> 32Bit_OneShot/2(CountTo)
  32Bit_OneShot/1(Done) -> rising edge/1(A)
  Inverter/1 -> 32Bit_OneShot/3(RST)  "output synched"
  rising edge/1(Q) -> Register/2
  Register/1 -> Logical/1, Out/1  "output"

== system volo_radio_controller/Shared Registers and IO Ports/There Can Only Be One ==
  A : Inport
  B : Inport  Port=2
  Inverter : xbsIndex_r4/Inverter  en=off  latency=0  dbl_ovrd=off  block_type=inv
  Inverter1 : xbsIndex_r4/Inverter  en=off  latency=0  dbl_ovrd=off  block_type=inv
  Logical1 : xbsIndex_r4/Logical  logical_function=AND  inputs=2  en=off  latency=0  precision=Full  arith_type=Unsigned  n_bits=16  bin_pt=0  align_bp=on  dbl_ovrd=off  block_type=logical
  Logical2 : xbsIndex_r4/Logical  logical_function=AND  inputs=2  en=off  latency=0  precision=Full  arith_type=Unsigned  n_bits=16  bin_pt=0  align_bp=on  dbl_ovrd=off  block_type=logical
  SafeA : Outport
  SafeB : Outport  Port=2
  wires:
  Logical1/1 -> SafeA/1
  Logical2/1 -> SafeB/1
  A/1 -> Logical1/1, Inverter1/1
  Inverter/1 -> Logical1/2
  B/1 -> Inverter/1, Logical2/2
  Inverter1/1 -> Logical2/1

== system volo_radio_controller/Shared Registers and IO Ports/negedge ==
  D : Inport
  Delay : xbsIndex_r4/Delay  rst=off  infoeditControl=Selection of Reset will increase slice count due to use of real FFs and instead of SRLs  en=off  latency=1  dbl_ovrd=off  reg_retiming=off  block_type=delay
      settings: infoedit=Hardware notes: A delay line is a chain, each link of which is an SRL16 followed by a flip-flop. If register retiming is enabled, the delay line is a chain of flip-flops.  xl_area=[1 1 0 0 0 0 0]  block_version=VER_STRING_GOES_HERE
  Inverter : xbsIndex_r4/Inverter  en=off  latency=0  dbl_ovrd=off  block_type=inv
      settings: xl_area=[0 0 0 0 0 0 0]  block_version=VER_STRING_GOES_HERE
  Logical1 : xbsIndex_r4/Logical  logical_function=AND  inputs=2  en=off  latency=0  precision=Full  arith_type=Unsigned  n_bits=8  bin_pt=2  align_bp=on  dbl_ovrd=off  block_type=logical
      settings: xl_area=[1 0 0 1 0 0 0]  block_version=VER_STRING_GOES_HERE
  Q : Outport
  wires:
  Delay/1 -> Logical1/2
  Logical1/1 -> Q/1
  D/1 -> Delay/1, Inverter/1
  Inverter/1 -> Logical1/1

== system volo_radio_controller/Shared Registers and IO Ports/negedge1 ==
  D : Inport
  Delay : xbsIndex_r4/Delay  rst=off  infoeditControl=Selection of Reset will increase slice count due to use of real FFs and instead of SRLs  en=off  latency=1  dbl_ovrd=off  reg_retiming=off  block_type=delay
      settings: infoedit=Hardware notes: A delay line is a chain, each link of which is an SRL16 followed by a flip-flop. If register retiming is enabled, the delay line is a chain of flip-flops.  xl_area=[1 1 0 0 0 0 0]  block_version=VER_STRING_GOES_HERE
  Inverter : xbsIndex_r4/Inverter  en=off  latency=0  dbl_ovrd=off  block_type=inv
      settings: xl_area=[0 0 0 0 0 0 0]  block_version=VER_STRING_GOES_HERE
  Logical1 : xbsIndex_r4/Logical  logical_function=AND  inputs=2  en=off  latency=0  precision=Full  arith_type=Unsigned  n_bits=8  bin_pt=2  align_bp=on  dbl_ovrd=off  block_type=logical
      settings: xl_area=[1 0 0 1 0 0 0]  block_version=VER_STRING_GOES_HERE
  Q : Outport
  wires:
  Delay/1 -> Logical1/2
  Logical1/1 -> Q/1
  D/1 -> Delay/1, Inverter/1
  Inverter/1 -> Logical1/1

== system volo_radio_controller/Shared Registers and IO Ports/negedge2 ==
  D : Inport
  Delay : xbsIndex_r4/Delay  rst=off  infoeditControl=Selection of Reset will increase slice count due to use of real FFs and instead of SRLs  en=off  latency=1  dbl_ovrd=off  reg_retiming=off  block_type=delay
      settings: infoedit=Hardware notes: A delay line is a chain, each link of which is an SRL16 followed by a flip-flop. If register retiming is enabled, the delay line is a chain of flip-flops.  xl_area=[1 1 0 0 0 0 0]  block_version=VER_STRING_GOES_HERE
  Inverter : xbsIndex_r4/Inverter  en=off  latency=0  dbl_ovrd=off  block_type=inv
      settings: xl_area=[0 0 0 0 0 0 0]  block_version=VER_STRING_GOES_HERE
  Logical1 : xbsIndex_r4/Logical  logical_function=AND  inputs=2  en=off  latency=0  precision=Full  arith_type=Unsigned  n_bits=8  bin_pt=2  align_bp=on  dbl_ovrd=off  block_type=logical
      settings: xl_area=[1 0 0 1 0 0 0]  block_version=VER_STRING_GOES_HERE
  Q : Outport
  wires:
  Delay/1 -> Logical1/2
  Logical1/1 -> Q/1
  D/1 -> Delay/1, Inverter/1
  Inverter/1 -> Logical1/1

== system volo_radio_controller/Shared Registers and IO Ports/posedge ==
  D : Inport
  Delay : xbsIndex_r4/Delay  rst=off  infoeditControl=Selection of Reset will increase slice count due to use of real FFs and instead of SRLs  en=off  latency=1  dbl_ovrd=off  reg_retiming=off  block_type=delay
      settings: infoedit=Hardware notes: A delay line is a chain, each link of which is an SRL16 followed by a flip-flop. If register retiming is enabled, the delay line is a chain of flip-flops.  xl_area=[1 1 0 0 0 0 0]  block_version=VER_STRING_GOES_HERE
  Inverter : xbsIndex_r4/Inverter  en=off  latency=0  dbl_ovrd=off  block_type=inv
      settings: xl_area=[0 0 0 0 0 0 0]  block_version=VER_STRING_GOES_HERE
  Logical1 : xbsIndex_r4/Logical  logical_function=AND  inputs=2  en=off  latency=0  precision=Full  arith_type=Unsigned  n_bits=8  bin_pt=2  align_bp=on  dbl_ovrd=off  block_type=logical
      settings: xl_area=[1 0 0 1 0 0 0]  block_version=VER_STRING_GOES_HERE
  Q : Outport
  wires:
  Inverter/1 -> Logical1/1
  D/1 -> Logical1/2, Delay/1
  Delay/1 -> Inverter/1
  Logical1/1 -> Q/1

== system volo_radio_controller/Shared Registers and IO Ports/posedge1 ==
  D : Inport
  Delay : xbsIndex_r4/Delay  rst=off  infoeditControl=Selection of Reset will increase slice count due to use of real FFs and instead of SRLs  en=off  latency=1  dbl_ovrd=off  reg_retiming=off  block_type=delay
      settings: infoedit=Hardware notes: A delay line is a chain, each link of which is an SRL16 followed by a flip-flop. If register retiming is enabled, the delay line is a chain of flip-flops.  xl_area=[1 1 0 0 0 0 0]  block_version=VER_STRING_GOES_HERE
  Inverter : xbsIndex_r4/Inverter  en=off  latency=0  dbl_ovrd=off  block_type=inv
      settings: xl_area=[0 0 0 0 0 0 0]  block_version=VER_STRING_GOES_HERE
  Logical1 : xbsIndex_r4/Logical  logical_function=AND  inputs=2  en=off  latency=0  precision=Full  arith_type=Unsigned  n_bits=8  bin_pt=2  align_bp=on  dbl_ovrd=off  block_type=logical
      settings: xl_area=[1 0 0 1 0 0 0]  block_version=VER_STRING_GOES_HERE
  Q : Outport
  wires:
  Inverter/1 -> Logical1/1
  D/1 -> Logical1/2, Delay/1
  Delay/1 -> Inverter/1
  Logical1/1 -> Q/1

== system volo_radio_controller/Shared Registers and IO Ports/posedge2 ==
  D : Inport
  Delay : xbsIndex_r4/Delay  rst=off  infoeditControl=Selection of Reset will increase slice count due to use of real FFs and instead of SRLs  en=off  latency=1  dbl_ovrd=off  reg_retiming=off  block_type=delay
      settings: infoedit=Hardware notes: A delay line is a chain, each link of which is an SRL16 followed by a flip-flop. If register retiming is enabled, the delay line is a chain of flip-flops.  xl_area=[1 1 0 0 0 0 0]  block_version=VER_STRING_GOES_HERE
  Inverter : xbsIndex_r4/Inverter  en=off  latency=0  dbl_ovrd=off  block_type=inv
      settings: xl_area=[0 0 0 0 0 0 0]  block_version=VER_STRING_GOES_HERE
  Logical1 : xbsIndex_r4/Logical  logical_function=AND  inputs=2  en=off  latency=0  precision=Full  arith_type=Unsigned  n_bits=8  bin_pt=2  align_bp=on  dbl_ovrd=off  block_type=logical
      settings: xl_area=[1 0 0 1 0 0 0]  block_version=VER_STRING_GOES_HERE
  Q : Outport
  wires:
  Inverter/1 -> Logical1/1
  D/1 -> Logical1/2, Delay/1
  Delay/1 -> Inverter/1
  Logical1/1 -> Q/1

== system volo_radio_controller/Shared Registers and IO Ports/RX Switching Delay/32Bit_OneShot ==
  Start : Inport
  CountTo : Inport  Port=2
  RST : Inport  Port=3
  HoldUntilReset : Subsystem
  Inverter2 : xbsIndex_r4/Inverter  en=off  latency=0  dbl_ovrd=off  block_type=inv
  Logical5 : xbsIndex_r4/Logical  logical_function=AND  inputs=2  en=off  latency=0  precision=Full  arith_type=Unsigned  n_bits=16  bin_pt=0  align_bp=on  dbl_ovrd=off  block_type=logical
  PayloadTimeoutCounter : xbsIndex_r4/Counter  cnt_type=Free Running  cnt_to=Inf  operation=Up  start_count=0  cnt_by_val=1  arith_type=Unsigned  n_bits=32  bin_pt=0  load_pin=off  rst=on  en=on  explicit_period=on  period=1  dbl_ovrd=off  use_behavioral_HDL=off  implementation=Fabric  block_type=counter
  Relational2 : xbsIndex_r4/Relational  mode=a=b  en=off  latency=0  dbl_ovrd=off  block_type=relational
  Done : Outport
  wires:
  RST/1 -> HoldUntilReset/2(RST), PayloadTimeoutCounter/1
  CountTo/1 -> Relational2/2
  PayloadTimeoutCounter/1 -> Relational2/1
  Relational2/1 -> Inverter2/1, Done/1  "payloadTimeout"
  Inverter2/1 -> Logical5/2
  Logical5/1 -> PayloadTimeoutCounter/2
  Start/1 -> HoldUntilReset/1(A)
  HoldUntilReset/1(Q) -> Logical5/1
